simulink model "tuning"  (R2023b)
settings: Solver=FixedStepAuto  StartTime=0.0  StopTime=10.0  RelTol=1e-3  EnableMultiTasking=on
values from neighbouring files (symbols this model uses):
  Ts = 0.005    [attempt.m]    (also in model_approximation.m; tuning.m)
libraries: mbedblockslib x3, stm_qeplib x1
settings Model: ExtModeTrigDuration=10  Creator=giova  LastModifiedBy=giova
settings OptimizationCC: EnhancedBackFolding=on  PassReuseOutputArgsAs=Individual arguments  ZeroExternalMemoryAtStartup=off  ZeroInternalMemoryAtStartup=off  MaxStackSize=64  OptimizeBlockOrder=speed  DifferentSizesBufferReuse=on  OptimizationCustomize=off  EfficientTunableParamExpr=on
settings DebuggingCC: ParameterTunabilityLossMsg=error
settings HardwareCC: ProdBitPerPointer=32  ProdBitPerSizeT=32  ProdBitPerPtrDiffT=32  ProdLargestAtomicInteger=Long  ProdLargestAtomicFloat=Double  ProdWordSize=32  ProdLongLongMode=on  ProdHWDeviceType=ARM Compatible->ARM Cortex
settings SFSimCC: MATLABDynamicMemAlloc=off
settings RTWCC: Description=Embedded Coder  SystemTargetFile=ert.tlc  HardwareBoard=STM32 Nucleo F401RE  TemplateMakefile=ert_default_tmf  Toolchain=GNU Tools for ARM Embedded Processors
settings CodeAppCC: ForceParamTrailComments=on  IgnoreCustomStorageClasses=off  OperatorAnnotations=on  SimulinkDataObjDesc=on  SFDataObjDesc=on  InsertBlockDesc=on
settings ERTTargetCC: ExtModeTransport=3  ExtModeStaticAlloc=on  ExtModeStaticAllocSize=2000  ExtModeMexFile=ext_xcp  ExtModeIntrfLevel=Level2 - Open

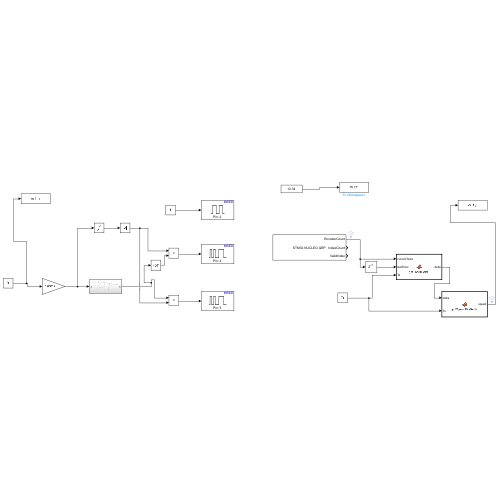
[thumbnail: Simulink's stored preview of the top-level diagram]
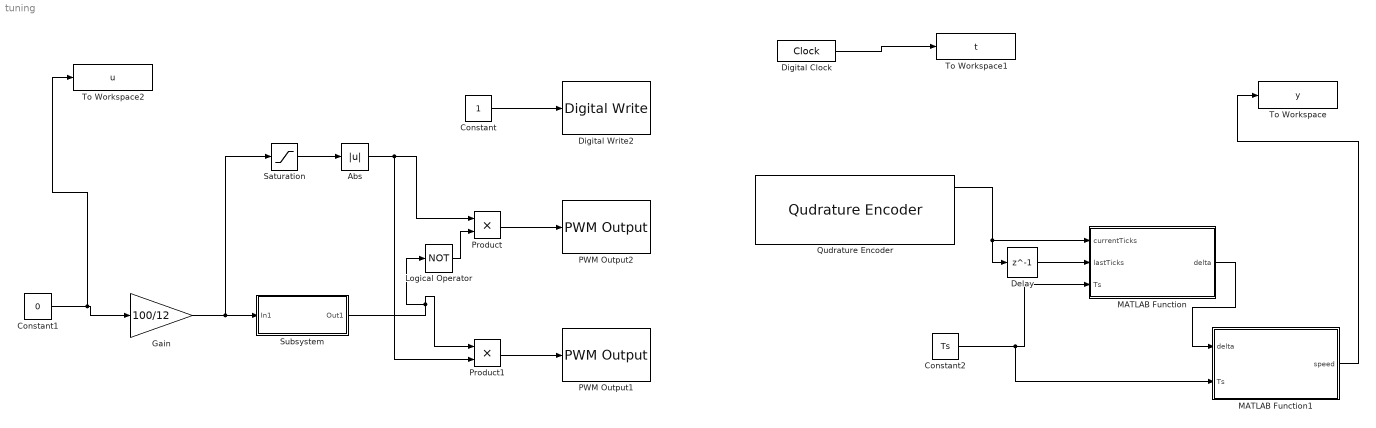
== system tuning ==
  Abs : Abs  SaturateOnIntegerOverflow=off
  Constant : Constant
  Constant1 : Constant  Value=0
  Constant2 : Constant  Value=Ts
  Delay : Delay  DelayLength=1  SampleTime=Ts
  Digital Clock : DigitalClock
  Digital Write2 : mbedblockslib/Digital Write  Pin=2  Direction=output
      settings: LibrarySourceBlock=stmnucleorootlib/Common/Digital Write
  Gain : Gain  Gain=100/12
  Logical Operator : Logic  Operator=NOT  AllPortsSameDT=off  OutDataTypeStr=boolean
  MATLAB Function : MATLAB Function  TreatAsAtomicUnit=on
  MATLAB Function1 : MATLAB Function  TreatAsAtomicUnit=on
  PWM Output1 : mbedblockslib/PWM Output  Pin=5  EnableInputFrequency=off  InitialFrequency=2000  InitialDutyCycle=50  NotificationType=None
      settings: LibrarySourceBlock=stmnucleorootlib/Common/PWM Output
  PWM Output2 : mbedblockslib/PWM Output  Pin=4  EnableInputFrequency=off  InitialFrequency=2000  InitialDutyCycle=50  NotificationType=None
      settings: LibrarySourceBlock=stmnucleorootlib/Common/PWM Output
  Product : Product
  Product1 : Product
  Qudrature Encoder : stm_qeplib/Qudrature Encoder  SampleTime=Ts
  Saturation : Saturate  UpperLimit=100  LowerLimit=-100
  Subsystem : Subsystem
  To Workspace : ToWorkspace  VariableName=y  SaveFormat=Timeseries  SampleTime=-1
  To Workspace1 : ToWorkspace  VariableName=t  SaveFormat=Timeseries  SampleTime=-1
  To Workspace2 : ToWorkspace  VariableName=u  SaveFormat=Timeseries  SampleTime=-1
  wires:
  Constant2/1 -> MATLAB Function1/2(Ts), MATLAB Function/3(Ts)
  Delay/1 -> MATLAB Function/2(lastTicks)
  Product/1 -> PWM Output2/1
  Subsystem/1(Out1) -> Logical Operator/1, Product1/1
  Product1/1 -> PWM Output1/1
  Qudrature Encoder/1 -> MATLAB Function/1(currentTicks), Delay/1
  Logical Operator/1 -> Product/2
  MATLAB Function/1(delta) -> MATLAB Function1/1(delta)
  Saturation/1 -> Abs/1
  Abs/1 -> Product1/2, Product/1
  Constant/1 -> Digital Write2/1
  MATLAB Function1/1(speed) -> To Workspace/1
  Constant1/1 -> To Workspace2/1, Gain/1
  Gain/1 -> Saturation/1, Subsystem/1(In1)
  Digital Clock/1 -> To Workspace1/1

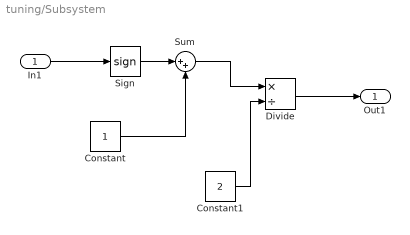
== system tuning/Subsystem ==
  In1 : Inport
  Constant : Constant
  Constant1 : Constant  Value=2
  Divide : Product  Inputs=*/
  Sign : Signum
  Sum : Sum  Inputs=|++
  Out1 : Outport
  wires:
  Constant/1 -> Sum/2
  In1/1 -> Sign/1
  Sign/1 -> Sum/1
  Sum/1 -> Divide/1
  Constant1/1 -> Divide/2
  Divide/1 -> Out1/1

== matlab function tuning/MATLAB Function ==
  data: currentTicks input; delta output; lastTicks input; Ts input
function delta = getTicksDelta(currentTicks, lastTicks, Ts)

currentTicks = double(currentTicks);
lastTicks = double(lastTicks);

if abs(currentTicks-lastTicks) <= ceil(12600*Ts)
    delta = currentTicks-lastTicks
else
    if lastTicks > currentTicks
        delta = currentTicks+2^16-1-lastTicks;
    else
        delta = currentTicks-2^16+1-lastTicks;
    end
end

end

== matlab function tuning/MATLAB Function1 ==
  data: delta input; speed output; Ts input
function speed = getSpeedByDelta(delta, Ts)
    speed = delta*60/(8400*Ts)

end
